simulink model "Math"  (R2017b)
settings: Solver=FixedStepAuto  StartTime=0.0  StopTime=10.0  FixedStep=0.1  RelTol=1e-3  EnableMultiTasking=on
undefined symbols (not defined in the file): magnitude
settings Model: Creator=ktrinh  LastModifiedBy=hbourbou
settings OptimizationCC: LifeSpan=inf
settings DebuggingCC: SFUnexpectedBacktrackingDiag=warning  SFNoUnconditionalDefaultTransitionDiag=warning  SFExecutionAtInitializationDiag=none
settings HardwareCC: ProdBitPerSizeT=32  ProdBitPerPtrDiffT=32  ProdWordSize=32  ProdHWDeviceType=Specified
settings CodeAppCC: StateflowObjectComments=on
settings GRTTargetCC: TargetLangStandard=C89/C90 (ANSI)  GeneratePreprocessorConditionals=Disable all
settings ConfigComp: CovMetricSettings=dw  CovHtmlReporting=on  CovSaveCumulativeToWorkspaceVar=on  CovSaveSingleToWorkspaceVar=on  CovExternalEMLEnable=off

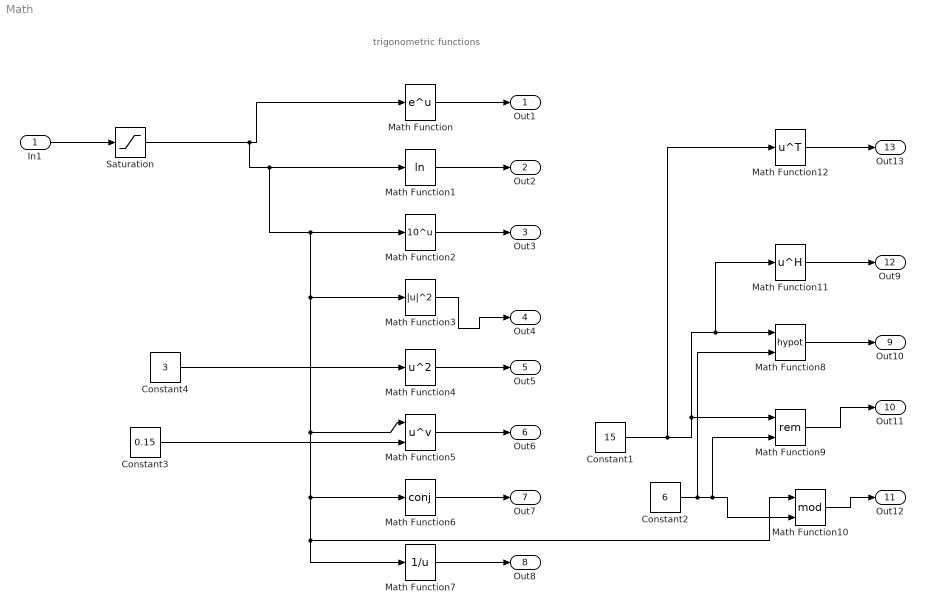
== system Math ==
  note: trigonometric functions
  In1 : Inport
  Constant1 : Constant  Value=15  OutDataTypeStr=double
  Constant2 : Constant  Value=6  OutDataTypeStr=double
  Constant3 : Constant  Value=0.15
  Constant4 : Constant  Value=3
  Math Function : Math  SaturateOnIntegerOverflow=on
  Math Function1 : Math  Operator=log  SaturateOnIntegerOverflow=on
  Math Function10 : Math  Operator=mod  SaturateOnIntegerOverflow=on
  Math Function11 : Math  Operator=hermitian  SaturateOnIntegerOverflow=on
  Math Function12 : Math  Operator=transpose  SaturateOnIntegerOverflow=on
  Math Function2 : Math  Operator=10^u  SaturateOnIntegerOverflow=on
  Math Function3 : Math  Operator=magnitude^2  SaturateOnIntegerOverflow=on
  Math Function4 : Math  Operator=square  OutDataTypeStr=int16  SaturateOnIntegerOverflow=on
  Math Function5 : Math  Operator=pow  SaturateOnIntegerOverflow=on
  Math Function6 : Math  Operator=conj  SaturateOnIntegerOverflow=on
  Math Function7 : Math  Operator=reciprocal  SaturateOnIntegerOverflow=on
  Math Function8 : Math  Operator=hypot  SaturateOnIntegerOverflow=on
  Math Function9 : Math  Operator=rem  SaturateOnIntegerOverflow=on
  Saturation : Saturate  UpperLimit=1.5  LowerLimit=0.5
  Out1 : Outport
  Out2 : Outport  Port=2
  Out3 : Outport  Port=3
  Out4 : Outport  Port=4
  Out5 : Outport  Port=5
  Out6 : Outport  Port=6
  Out7 : Outport  Port=7
  Out8 : Outport  Port=8
  Out10 : Outport  Port=9
  Out11 : Outport  Port=10
  Out12 : Outport  Port=11
  Out9 : Outport  Port=12
  Out13 : Outport  Port=13
  wires:
  Math Function/1 -> Out1/1
  Math Function1/1 -> Out2/1
  Math Function2/1 -> Out3/1
  Math Function3/1 -> Out4/1
  Math Function4/1 -> Out5/1
  Math Function5/1 -> Out6/1
  Math Function6/1 -> Out7/1
  Math Function7/1 -> Out8/1
  Saturation/1 -> Math Function/1, Math Function1/1, Math Function2/1, Math Function3/1, Math Function5/1, Math Function6/1, Math Function7/1, Math Function10/1
  Constant1/1 -> Math Function12/1, Math Function11/1, Math Function8/1, Math Function9/1
  Math Function9/1 -> Out11/1
  Math Function8/1 -> Out10/1
  Math Function10/1 -> Out12/1
  Math Function12/1 -> Out13/1
  Math Function11/1 -> Out9/1
  Constant2/1 -> Math Function8/2, Math Function9/2, Math Function10/2
  Constant3/1 -> Math Function5/2
  Constant4/1 -> Math Function4/1
  In1/1 -> Saturation/1
